simulink model "fulltry"  (R2023b)
settings: Solver=VariableStepAuto  StartTime=0.0  StopTime=40  RelTol=1e-3
undefined symbols (not defined in the file): C_dc, c_drt, C_p_opt, H_gen, H_vsm, H_WTR, I_dc_0, I_dc_base, Ibase_lv, k_d_vsm, k_drt, k_p_p_vsm, k_p_q_vsm, K_pitch, ki_q, L_d, l_f, L_grid, L_q, lambda_opt, Lbase1v, omega_nom, omega_WTR_min, omega_WTR_n, omega_WTR_sl, phase_shift_test_state, phase_shifts, pitch_max, pitch_min, Pitchanglevector, Pmax, Powercoefficient, psi_pm, R_a, r_f, R_grid, R_WTR, rate_max, rate_min, rocof_slope, Rocof_test_state, Sbase1, T_base, T_pitch, T_servo, Tchange_gfm_ref, Trocof_end, Trocof_start, Ts, TSRvector, V_dc, V_dc_base, v_w_n, Vbase_lv, voltage_sag_test_state, wind_array_step, Zbase1v
libraries: spsControlledVoltageSourceLib x6, spsPower3phInstantaneousLib x4, slpidlib x3, spsThreePhaseVIMeasurementLib x3, spsRMSLib x3, spsdq0toabcLib x2, spsCurrentMeasurementLib x2, spsSeriesRLCBranchLib x2, spsVoltageMeasurementLib x2, spsThreePhaseSeriesRLCBranchLib x2, spsDCVoltageSourceLib x2, spsGroundLib x1
(part 2 of 2)

== matlab function fulltry/Subsystem2/Aerodynamic power/CP_calculator ==
  data: Theta input; R_WTR input; omega_WTR input; cp output; U input; lambda output
function  [cp, lambda] = fcn(Theta,R_WTR,omega_WTR,U) 
    
    lambda = omega_WTR*R_WTR/U;

    c = [0.645 116 0.4 5 21 0.00912 0.08 0.035 0.001];
    a = (-c(4)-c(3)*(2.5+Theta)+c(2)*1/(lambda+c(7)*(2.5+Theta))-c(8)/(lambda+(2.5+Theta)^3));
    exponent = c(5)*1/(lambda+c(7)*(2.5+Theta))-c(8)/(lambda+(2.5+Theta)^3);
    x = c(1)*(c(6)*lambda+a/exp(exponent))+c(9)*lambda;

cp = x;
